simulink model "bus_test"  (Simulink 9.0)
settings: Solver=FixedStepAuto  StartTime=0.0  StopTime=10.0  FixedStep=0.1  RelTol=1e-3  EnableMultiTasking=on
undefined symbols (not defined in the file): signal1, signal3
settings Model: SuppressorTable=22 serialization::archive 11 0 6 0 0 0 0 0  Creator=arnaud  LastModifiedBy=hbourbou
settings DataIOCC: LimitDataPoints=on  SaveFormat=StructureWithTime  SignalLoggingSaveFormat=ModelDataLogs
settings OptimizationCC: ExpressionDepthLimit=2147483647
settings DebuggingCC: SolverPrmCheckMsg=warning  FcnCallInpInsideContextMsg=warning  StateNameClashWarn=warning
settings GRTTargetCC: GeneratePreprocessorConditionals=Disable all  CombineOutputUpdateFcns=off  GRTInterface=on
settings ConfigComp: CovSFcnEnable=off

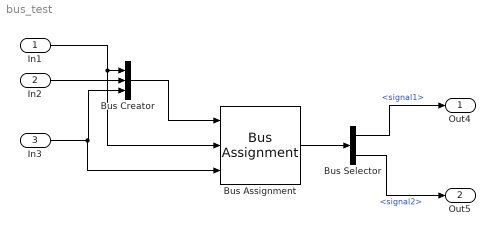
== system bus_test ==
  In1 : Inport  PortDimensions=1
  In2 : Inport  Port=2  OutDataTypeStr=int8  PortDimensions=2
  In3 : Inport  Port=3  OutDataTypeStr=boolean  PortDimensions=3
  Bus Assignment : BusAssignment  AssignedSignals=signal1,signal3
  Bus Creator : BusCreator  Inputs=3
  Bus Selector : BusSelector  OutputSignals=signal1,signal2
  Out4 : Outport
  Out5 : Outport  Port=2
  wires:
  In2/1 -> Bus Creator/2
  In3/1 -> Bus Assignment/3, Bus Creator/3
  In1/1 -> Bus Assignment/2, Bus Creator/1
  Bus Creator/1 -> Bus Assignment/1
  Bus Selector/1 -> Out4/1  "<signal1>"
  Bus Selector/2 -> Out5/1  "<signal2>"
  Bus Assignment/1 -> Bus Selector/1
